simulink model "amp2"  (R2025b)
settings: Solver=FixedStepDiscrete  StartTime=0.0  StopTime=inf  RelTol=1e-3
settings Model: Creator=linogarciamorales  LastModifiedBy=linogarciamorales
settings OptimizationCC: DefaultParameterBehavior=Inlined  EnhancedBackFolding=on  PassReuseOutputArgsAs=Individual arguments  ZeroExternalMemoryAtStartup=off  ZeroInternalMemoryAtStartup=off  OptimizeBlockOrder=speed  DifferentSizesBufferReuse=on  OptimizationCustomize=off  EfficientTunableParamExpr=on
settings DebuggingCC: ParameterTunabilityLossMsg=error
settings HardwareCC: ProdBitPerPointer=32.0  ProdBitPerSizeT=32.0  ProdBitPerPtrDiffT=32.0  ProdLargestAtomicInteger=Long  ProdLargestAtomicFloat=Double  ProdWordSize=32.0  ProdHWDeviceType=ARM Compatible->ARM Cortex-A  TargetLargestAtomicInteger=Long  TargetLargestAtomicFloat=Double  TargetIntDivRoundTo=Zero  TargetEndianess=LittleEndian  TargetHWDeviceType=ARM Compatible->ARM Cortex-A
settings SFSimCC: MATLABDynamicMemAlloc=off
settings RTWCC: SystemTargetFile=ert.tlc  GenCodeOnly=on  TemplateMakefile=ert_default_tmf  PortableWordSizes=on  Description=Embedded Coder
settings CodeAppCC: ForceParamTrailComments=on  IgnoreCustomStorageClasses=off  OperatorAnnotations=on  SimulinkDataObjDesc=on  SFDataObjDesc=on  InsertBlockDesc=on
settings ERTTargetCC: ERTCustomFileTemplate=example_file_process.tlc  TargetLangStandard=C99 (ISO)  GenerateSampleERTMain=on  SupportNonInlinedSFcns=on

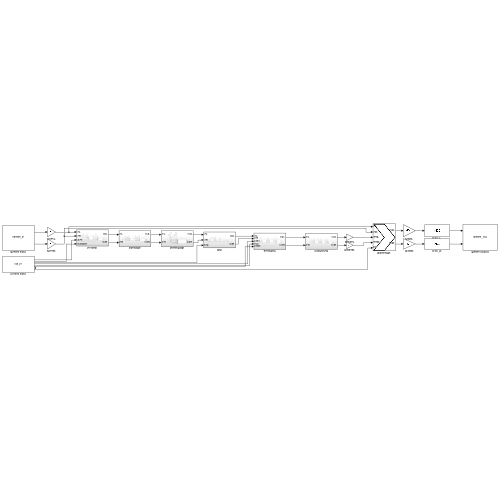
[thumbnail: Simulink's stored preview of the top-level diagram]
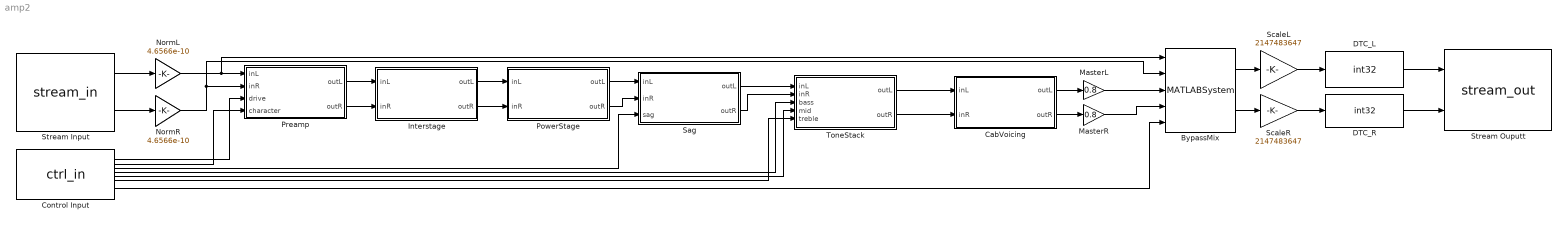
== system amp2 ==
  BypassMix : MATLABSystem  System=mix_sys  N=128  Fs=48000  Mode=uint8( 0 )  SmoothTime=0.02  IndepInDB=false  SimulateUsing=Code generation
      mask Type: mix_sys
  CabVoicing : Subsystem
  Control Input : S-Function  FunctionName=ctrl_in  Parameters=48000,128,8  SFunctionDeploymentMode=off  EnableBusSupport=off
  DTC_L : DataTypeConversion  OutDataTypeStr=int32  SaturateOnIntegerOverflow=off  RndMeth=Floor
  DTC_R : DataTypeConversion  OutDataTypeStr=int32  SaturateOnIntegerOverflow=off  RndMeth=Floor
  Interstage : Subsystem
  MasterL : Gain  Gain=0.8
  MasterR : Gain  Gain=0.8
  NormL : Gain  Gain=4.6566e-10  OutDataTypeStr=double
  NormR : Gain  Gain=4.6566e-10  OutDataTypeStr=double
  PowerStage : Subsystem
  Preamp : Subsystem
  Sag : Subsystem
  ScaleL : Gain  Gain=2147483647
  ScaleR : Gain  Gain=2147483647
  Stream Input : S-Function  FunctionName=stream_in  Parameters=48000,128,0  SFunctionDeploymentMode=off  EnableBusSupport=off
  Stream Ouputt : S-Function  FunctionName=stream_out  Parameters=48000,128,0  SFunctionDeploymentMode=off  EnableBusSupport=off
  ToneStack : Subsystem
  wires:
  Stream Input/1 -> NormL/1
  Stream Input/2 -> NormR/1
  Control Input/1 -> Preamp/3(drive)
  Control Input/2 -> Preamp/4(character)
  Control Input/3 -> Sag/3(sag)
  Control Input/4 -> ToneStack/3(bass)
  Control Input/5 -> ToneStack/4(mid)
  Control Input/6 -> ToneStack/5(treble)
  Preamp/1(outL) -> Interstage/1(inL)
  Preamp/2(outR) -> Interstage/2(inR)
  Interstage/1(outL) -> PowerStage/1(inL)
  Interstage/2(outR) -> PowerStage/2(inR)
  PowerStage/1(outL) -> Sag/1(inL)
  PowerStage/2(outR) -> Sag/2(inR)
  Sag/1(outL) -> ToneStack/1(inL)
  Sag/2(outR) -> ToneStack/2(inR)
  ToneStack/1(outL) -> CabVoicing/1(inL)
  ToneStack/2(outR) -> CabVoicing/2(inR)
  DTC_L/1 -> Stream Ouputt/1
  DTC_R/1 -> Stream Ouputt/2
  ScaleR/1 -> DTC_R/1
  ScaleL/1 -> DTC_L/1
  BypassMix/2 -> ScaleR/1
  BypassMix/1 -> ScaleL/1
  Control Input/8 -> BypassMix/5
  MasterR/1 -> BypassMix/4
  MasterL/1 -> BypassMix/3
  CabVoicing/2(outR) -> MasterR/1
  CabVoicing/1(outL) -> MasterL/1
  NormR/1 -> BypassMix/2, Preamp/2(inR)
  NormL/1 -> BypassMix/1, Preamp/1(inL)

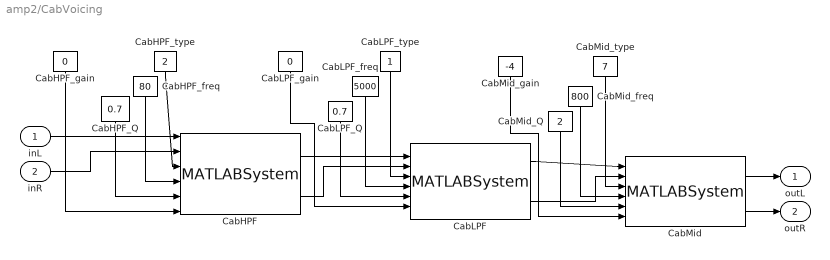
== system amp2/CabVoicing ==
  inL : Inport
  inR : Inport  Port=2
  CabHPF : MATLABSystem  System=vcf_sys  N=128  Fs=48000  bypass=uint8(0)  SimulateUsing=Code generation
      mask Type: vcf_sys
  CabHPF_Q : Constant  Value=0.7
  CabHPF_freq : Constant  Value=80
  CabHPF_gain : Constant  Value=0
  CabHPF_type : Constant  Value=2
  CabLPF : MATLABSystem  System=vcf_sys  N=128  Fs=48000  bypass=uint8(0)  SimulateUsing=Code generation
      mask Type: vcf_sys
  CabLPF_Q : Constant  Value=0.7
  CabLPF_freq : Constant  Value=5000
  CabLPF_gain : Constant  Value=0
  CabLPF_type : Constant
  CabMid : MATLABSystem  System=vcf_sys  N=128  Fs=48000  bypass=uint8(0)  SimulateUsing=Code generation
      mask Type: vcf_sys
  CabMid_Q : Constant  Value=2
  CabMid_freq : Constant  Value=800
  CabMid_gain : Constant  Value=-4
  CabMid_type : Constant  Value=7
  outL : Outport
  outR : Outport  Port=2
  wires:
  inL/1 -> CabHPF/1
  inR/1 -> CabHPF/2
  CabHPF_type/1 -> CabHPF/3
  CabHPF_freq/1 -> CabHPF/4
  CabHPF_Q/1 -> CabHPF/5
  CabHPF_gain/1 -> CabHPF/6
  CabHPF/1 -> CabLPF/1
  CabHPF/2 -> CabLPF/2
  CabLPF_type/1 -> CabLPF/3
  CabLPF_freq/1 -> CabLPF/4
  CabLPF_Q/1 -> CabLPF/5
  CabLPF_gain/1 -> CabLPF/6
  CabLPF/1 -> CabMid/1
  CabLPF/2 -> CabMid/2
  CabMid_type/1 -> CabMid/3
  CabMid_freq/1 -> CabMid/4
  CabMid_Q/1 -> CabMid/5
  CabMid_gain/1 -> CabMid/6
  CabMid/1 -> outL/1
  CabMid/2 -> outR/1

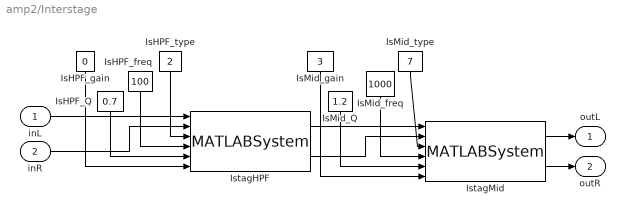
== system amp2/Interstage ==
  inL : Inport
  inR : Inport  Port=2
  IsHPF_Q : Constant  Value=0.7
  IsHPF_freq : Constant  Value=100
  IsHPF_gain : Constant  Value=0
  IsHPF_type : Constant  Value=2
  IsMid_Q : Constant  Value=1.2
  IsMid_freq : Constant  Value=1000
  IsMid_gain : Constant  Value=3
  IsMid_type : Constant  Value=7
  IstagHPF : MATLABSystem  System=vcf_sys  N=128  Fs=48000  bypass=uint8(0)  SimulateUsing=Code generation
      mask Type: vcf_sys
  IstagMid : MATLABSystem  System=vcf_sys  N=128  Fs=48000  bypass=uint8(0)  SimulateUsing=Code generation
      mask Type: vcf_sys
  outL : Outport
  outR : Outport  Port=2
  wires:
  inL/1 -> IstagHPF/1
  inR/1 -> IstagHPF/2
  IsHPF_type/1 -> IstagHPF/3
  IsHPF_freq/1 -> IstagHPF/4
  IsHPF_Q/1 -> IstagHPF/5
  IsHPF_gain/1 -> IstagHPF/6
  IstagHPF/1 -> IstagMid/1
  IstagHPF/2 -> IstagMid/2
  IsMid_type/1 -> IstagMid/3
  IsMid_freq/1 -> IstagMid/4
  IsMid_Q/1 -> IstagMid/5
  IsMid_gain/1 -> IstagMid/6
  IstagMid/1 -> outL/1
  IstagMid/2 -> outR/1

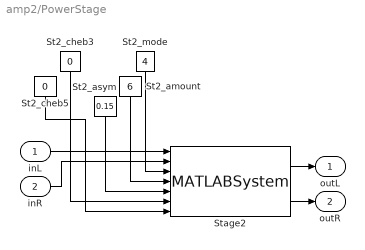
== system amp2/PowerStage ==
  inL : Inport
  inR : Inport  Port=2
  St2_amount : Constant  Value=6
  St2_asym : Constant  Value=0.15
  St2_cheb3 : Constant  Value=0
  St2_cheb5 : Constant  Value=0
  St2_mode : Constant  Value=4
  Stage2 : MATLABSystem  System=lut_ws_sys  N=128  M=257  bypass=uint8(0)  OS=uint8(0)  HB15=[ -1.06360599e-04, 0, 6.95210045e-03, 0, -5.16884606e-02, 0, 2.94825487e-01, 5.00034468e-01, 2.94825487e-01, 0, -5.16884606e-02, 0, 6.95210045e-03, 0, -1.06360599e-04 ]  ModeDefault=uint8( 3 )  AmountDefault=12.0  AsymDefault=0.0  Cheb3Default=1.0  Cheb5Default=0.0  XUser=linspace( -1, 1, 257 )  YUser=linspace( -1, 1, 257 )  MUser=257  Eps=1e-12  SimulateUsing=Code generation
      mask Type: lut_ws_sys
  outL : Outport
  outR : Outport  Port=2
  wires:
  inL/1 -> Stage2/1
  inR/1 -> Stage2/2
  St2_mode/1 -> Stage2/3
  St2_amount/1 -> Stage2/4
  St2_asym/1 -> Stage2/5
  St2_cheb3/1 -> Stage2/6
  St2_cheb5/1 -> Stage2/7
  Stage2/1 -> outL/1
  Stage2/2 -> outR/1

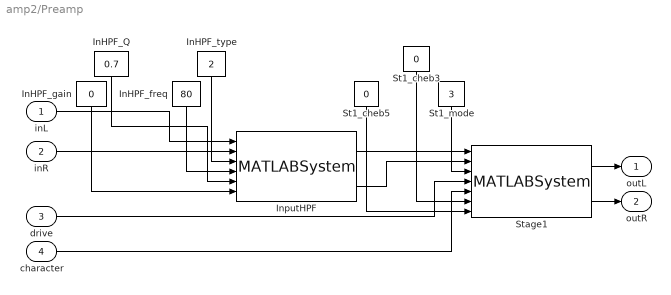
== system amp2/Preamp ==
  inL : Inport
  inR : Inport  Port=2
  drive : Inport  Port=3
  character : Inport  Port=4
  InHPF_Q : Constant  Value=0.7
  InHPF_freq : Constant  Value=80
  InHPF_gain : Constant  Value=0
  InHPF_type : Constant  Value=2
  InputHPF : MATLABSystem  System=vcf_sys  N=128  Fs=48000  bypass=uint8(0)  SimulateUsing=Code generation
      mask Type: vcf_sys
  St1_cheb3 : Constant  Value=0
  St1_cheb5 : Constant  Value=0
  St1_mode : Constant  Value=3
  Stage1 : MATLABSystem  System=lut_ws_sys  N=128  M=257  bypass=uint8(0)  OS=uint8(0)  HB15=[ -1.06360599e-04, 0, 6.95210045e-03, 0, -5.16884606e-02, 0, 2.94825487e-01, 5.00034468e-01, 2.94825487e-01, 0, -5.16884606e-02, 0, 6.95210045e-03, 0, -1.06360599e-04 ]  ModeDefault=uint8( 3 )  AmountDefault=12.0  AsymDefault=0.0  Cheb3Default=1.0  Cheb5Default=0.0  XUser=linspace( -1, 1, 257 )  YUser=linspace( -1, 1, 257 )  MUser=257  Eps=1e-12  SimulateUsing=Code generation
      mask Type: lut_ws_sys
  outL : Outport
  outR : Outport  Port=2
  wires:
  inL/1 -> InputHPF/1
  inR/1 -> InputHPF/2
  InHPF_type/1 -> InputHPF/3
  InHPF_freq/1 -> InputHPF/4
  InHPF_Q/1 -> InputHPF/5
  InHPF_gain/1 -> InputHPF/6
  InputHPF/1 -> Stage1/1
  InputHPF/2 -> Stage1/2
  drive/1 -> Stage1/4
  character/1 -> Stage1/5
  St1_cheb3/1 -> Stage1/6
  St1_cheb5/1 -> Stage1/7
  Stage1/1 -> outL/1
  Stage1/2 -> outR/1
  St1_mode/1 -> Stage1/3

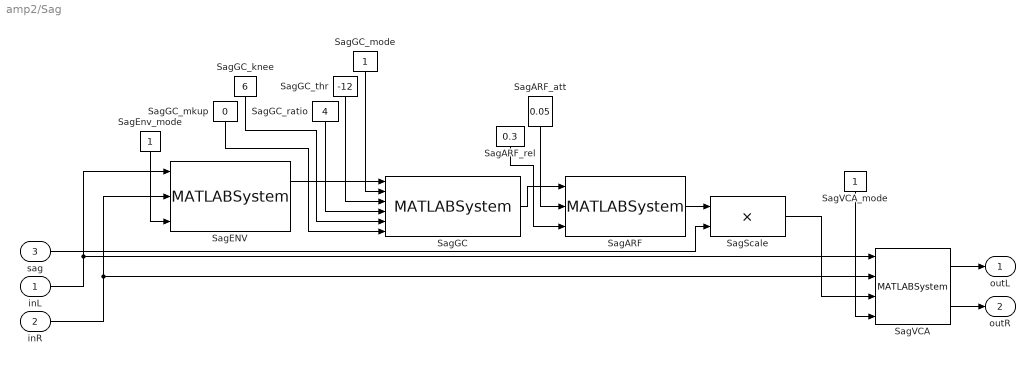
== system amp2/Sag ==
  inL : Inport
  inR : Inport  Port=2
  sag : Inport  Port=3
  SagARF : MATLABSystem  System=arf_sys  N=128  Fs=48000  bypass=uint8(0)  SimulateUsing=Code generation
      mask Type: arf_sys
  SagARF_att : Constant  Value=0.05
  SagARF_rel : Constant  Value=0.3
  SagENV : MATLABSystem  System=env_sys  N=128  Fs=48000  ModeDefault=uint8( 1 )  Eps=1e-12  TauRMS=0.02  SimulateUsing=Code generation
      mask Type: env_sys
  SagEnv_mode : Constant
  SagGC : MATLABSystem  System=lut_gc_sys  N=128  Fs=48000  M=257  Xmin=-80  Xmax=10  Floor_dB=-80  XUser=linspace( -80, 10, 257 )  YUser=zeros( 1, 257 )  MUser=257  SimulateUsing=Code generation
      mask Type: lut_gc_sys
  SagGC_knee : Constant  Value=6
  SagGC_mkup : Constant  Value=0
  SagGC_mode : Constant
  SagGC_ratio : Constant  Value=4
  SagGC_thr : Constant  Value=-12
  SagScale : Product  Inputs=**
  SagVCA : MATLABSystem  System=vca_sys  N=128  Fs=48000  bypass=uint8(0)  SimulateUsing=Code generation
      mask Type: vca_sys
  SagVCA_mode : Constant
  outL : Outport
  outR : Outport  Port=2
  wires:
  inL/1 -> SagENV/1, SagVCA/1
  inR/1 -> SagENV/2, SagVCA/2
  SagEnv_mode/1 -> SagENV/3
  SagENV/1 -> SagGC/1
  SagGC_mode/1 -> SagGC/2
  SagGC_thr/1 -> SagGC/3
  SagGC_ratio/1 -> SagGC/4
  SagGC_knee/1 -> SagGC/5
  SagGC_mkup/1 -> SagGC/6
  SagGC/1 -> SagARF/1
  SagARF_att/1 -> SagARF/2
  SagARF_rel/1 -> SagARF/3
  SagARF/1 -> SagScale/1
  sag/1 -> SagScale/2
  SagScale/1 -> SagVCA/3
  SagVCA_mode/1 -> SagVCA/4
  SagVCA/1 -> outL/1
  SagVCA/2 -> outR/1

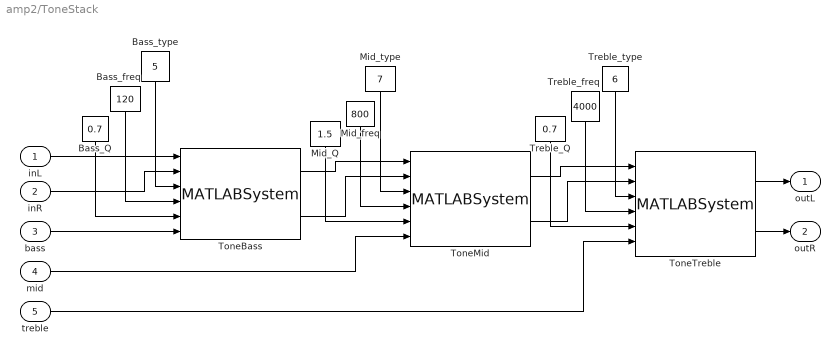
== system amp2/ToneStack ==
  inL : Inport
  inR : Inport  Port=2
  bass : Inport  Port=3
  mid : Inport  Port=4
  treble : Inport  Port=5
  Bass_Q : Constant  Value=0.7
  Bass_freq : Constant  Value=120
  Bass_type : Constant  Value=5
  Mid_Q : Constant  Value=1.5
  Mid_freq : Constant  Value=800
  Mid_type : Constant  Value=7
  ToneBass : MATLABSystem  System=vcf_sys  N=128  Fs=48000  bypass=uint8(0)  SimulateUsing=Code generation
      mask Type: vcf_sys
  ToneMid : MATLABSystem  System=vcf_sys  N=128  Fs=48000  bypass=uint8(0)  SimulateUsing=Code generation
      mask Type: vcf_sys
  ToneTreble : MATLABSystem  System=vcf_sys  N=128  Fs=48000  bypass=uint8(0)  SimulateUsing=Code generation
      mask Type: vcf_sys
  Treble_Q : Constant  Value=0.7
  Treble_freq : Constant  Value=4000
  Treble_type : Constant  Value=6
  outL : Outport
  outR : Outport  Port=2
  wires:
  inL/1 -> ToneBass/1
  inR/1 -> ToneBass/2
  Bass_type/1 -> ToneBass/3
  Bass_freq/1 -> ToneBass/4
  Bass_Q/1 -> ToneBass/5
  bass/1 -> ToneBass/6
  ToneBass/1 -> ToneMid/1
  ToneBass/2 -> ToneMid/2
  Mid_type/1 -> ToneMid/3
  Mid_freq/1 -> ToneMid/4
  Mid_Q/1 -> ToneMid/5
  mid/1 -> ToneMid/6
  ToneMid/1 -> ToneTreble/1
  ToneMid/2 -> ToneTreble/2
  Treble_type/1 -> ToneTreble/3
  Treble_freq/1 -> ToneTreble/4
  Treble_Q/1 -> ToneTreble/5
  treble/1 -> ToneTreble/6
  ToneTreble/1 -> outL/1
  ToneTreble/2 -> outR/1
